simulink model "scheme2"  (R2014a)
settings: Solver=ode45  StartTime=0.0  StopTime=0.4  RelTol=1e-3
settings Model: Creator=User  LastModifiedBy=trigg

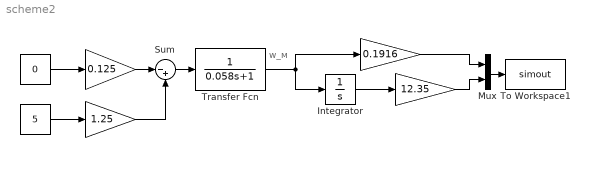
== system scheme2 ==
  note: w_м
  " " : Gain  Gain=1.25
  "  " : Constant  Value=5
  "   " : Constant  Value=0
  "    " : Gain  Gain=0.125
  "     " : Gain  Gain=0.1916
  "       " : Gain  Gain=12.35
  Integrator : Integrator
  Mux : Mux  Inputs=2
  Sum : Sum  Inputs=|-+
  To Workspace1 : ToWorkspace  VariableName=simout  SaveFormat=Timeseries  SampleTime=-1
  Transfer Fcn : TransferFcn  Denominator=[0.058 1]
  wires:
  Sum/1 -> Transfer Fcn/1
  Integrator/1 -> "       "/1
  "  "/1 -> " "/1
  "   "/1 -> "    "/1
  " "/1 -> Sum/2
  "    "/1 -> Sum/1
  "     "/1 -> Mux/1
  "       "/1 -> Mux/2
  Mux/1 -> To Workspace1/1
  Transfer Fcn/1 -> "     "/1, Integrator/1
